simulink model "log_map_sl"  (Simulink 7.5)
settings: Solver=FixedStepDiscrete  StartTime=0.0  StopTime=50.0  FixedStep=0.1  RelTol=1e-3
values from neighbouring files (symbols this model uses):
  alpha = 0.2    [logmap_start.m]
  beta = 0.7    [logmap_start.m]
  lambda = 4.0    (= 4)    [logmap_start.m]
  y1_0 = 0.23421    [logmap_start.m]
  y2_0 = 0.86567    [logmap_start.m]
settings Model: OSC_ATGCV_WORKDIR=C:\test_ground\target_link_stuff\sixth\new_profile  Creator=alex  LastModifiedBy=alex
settings DataIOCC: LimitDataPoints=off  SaveOutput=off  SaveTime=off
settings OptimizationCC: BooleanDataType=off  InitFltsAndDblsToZero=on
settings DebuggingCC: SaveWithParameterizedLinksMsg=none  SignalResolutionControl=TryResolveAllWithWarning  SolverPrmCheckMsg=none  MultiTaskDSMMsg=warning  MultiTaskCondExecSysMsg=none  StrictBusMsg=None
settings HardwareCC: TargetUnknown=on
settings RTWCC: IncludeERTFirstTime=on
settings GRTTargetCC: TargetFcnLib=ansi_tfl_tmw.mat

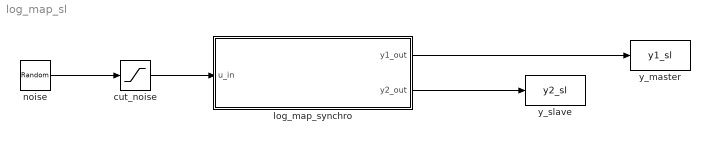
== system log_map_sl ==
  cut_noise : Saturate  UpperLimit=1  LowerLimit=0
  log_map_synchro : Subsystem
  noise : RandomNumber  Mean=0.5  SampleTime=0
  y_master : ToWorkspace  VariableName=y1_sl  SampleTime=-1  SaveFormat=Array
  y_slave : ToWorkspace  VariableName=y2_sl  SampleTime=-1  SaveFormat=Array
  wires:
  noise/1 -> cut_noise/1
  log_map_synchro/1(y1_out) -> y_master/1
  cut_noise/1 -> log_map_synchro/1(u_in)
  log_map_synchro/2(y2_out) -> y_slave/1

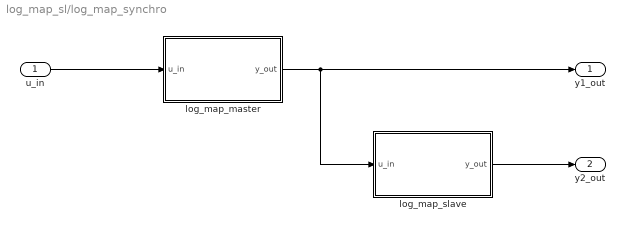
== system log_map_sl/log_map_synchro ==
  u_in : Inport  OutDataType=sfix(16)  OutScaling=2^0
  log_map_master : Subsystem
  log_map_slave : Subsystem
  y1_out : Outport  OutDataType=sfix(16)  OutScaling=2^0
  y2_out : Outport  Port=2  OutDataType=sfix(16)  OutScaling=2^0
  wires:
  u_in/1 -> log_map_master/1(u_in)
  log_map_master/1(y_out) -> y1_out/1, log_map_slave/1(u_in)
  log_map_slave/1(y_out) -> y2_out/1

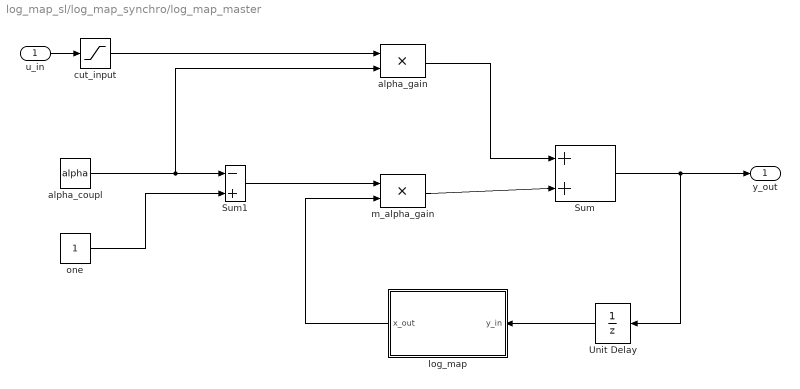
== system log_map_sl/log_map_synchro/log_map_master ==
  u_in : Inport  OutDataType=sfix(16)  OutScaling=2^0
  Sum : Sum  Inputs=+|+  OutDataType=sfix(16)  OutScaling=2^0  SaturateOnIntegerOverflow=on  InputSameDT=on  OutDataTypeStr=Inherit: Same as first input
  Sum1 : Sum  Inputs=-|+  OutDataType=sfix(16)  OutScaling=2^0  SaturateOnIntegerOverflow=on  InputSameDT=on  OutDataTypeStr=Inherit: Same as first input
  Unit Delay : UnitDelay  X0=y1_0  SampleTime=-1
  alpha_coupl : Constant  Value=alpha  OutDataType=sfix(16)  OutScaling=2^0
  alpha_gain : Product  OutDataType=sfix(16)  OutScaling=2^0  SaturateOnIntegerOverflow=on  RndMeth=Zero  InputSameDT=on  OutDataTypeStr=Inherit: Same as first input
  cut_input : Saturate  UpperLimit=1  LowerLimit=0
  log_map : Subsystem
  m_alpha_gain : Product  OutDataType=sfix(16)  OutScaling=2^0  SaturateOnIntegerOverflow=on  RndMeth=Zero  InputSameDT=on  OutDataTypeStr=Inherit: Same as first input
  one : Constant  OutDataType=sfix(16)  OutScaling=2^0
  y_out : Outport  OutDataType=sfix(16)  OutScaling=2^0
  wires:
  alpha_gain/1 -> Sum/1
  log_map/1(x_out) -> m_alpha_gain/2
  Sum/1 -> Unit Delay/1, y_out/1
  u_in/1 -> cut_input/1
  cut_input/1 -> alpha_gain/1
  Unit Delay/1 -> log_map/1(y_in)
  m_alpha_gain/1 -> Sum/2
  one/1 -> Sum1/2
  alpha_coupl/1 -> Sum1/1, alpha_gain/2
  Sum1/1 -> m_alpha_gain/1

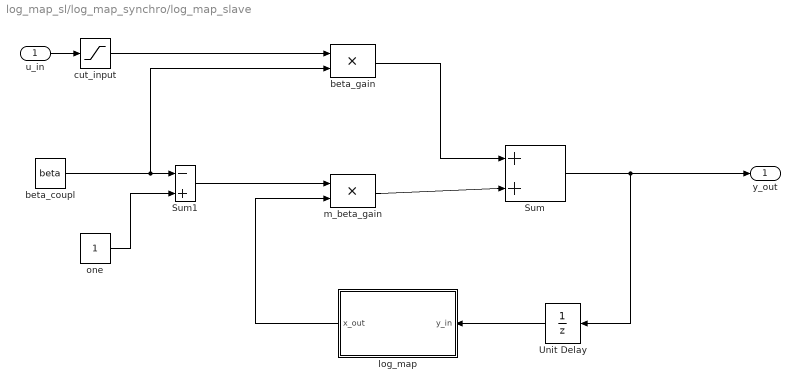
== system log_map_sl/log_map_synchro/log_map_slave ==
  u_in : Inport  OutDataType=sfix(16)  OutScaling=2^0
  Sum : Sum  Inputs=+|+  OutDataType=sfix(16)  OutScaling=2^0  SaturateOnIntegerOverflow=on  InputSameDT=on  OutDataTypeStr=Inherit: Same as first input
  Sum1 : Sum  Inputs=-|+  OutDataType=sfix(16)  OutScaling=2^0  SaturateOnIntegerOverflow=on  InputSameDT=on  OutDataTypeStr=Inherit: Same as first input
  Unit Delay : UnitDelay  X0=y2_0  SampleTime=-1
  beta_coupl : Constant  Value=beta  OutDataType=sfix(16)  OutScaling=2^0
  beta_gain : Product  OutDataType=sfix(16)  OutScaling=2^0  SaturateOnIntegerOverflow=on  RndMeth=Zero  InputSameDT=on  OutDataTypeStr=Inherit: Same as first input
  cut_input : Saturate  UpperLimit=1  LowerLimit=0
  log_map : Subsystem
  m_beta_gain : Product  OutDataType=sfix(16)  OutScaling=2^0  SaturateOnIntegerOverflow=on  RndMeth=Zero  InputSameDT=on  OutDataTypeStr=Inherit: Same as first input
  one : Constant  OutDataType=sfix(16)  OutScaling=2^0
  y_out : Outport  OutDataType=sfix(16)  OutScaling=2^0
  wires:
  m_beta_gain/1 -> Sum/2
  Unit Delay/1 -> log_map/1(y_in)
  cut_input/1 -> beta_gain/1
  u_in/1 -> cut_input/1
  Sum/1 -> y_out/1, Unit Delay/1
  log_map/1(x_out) -> m_beta_gain/2
  beta_gain/1 -> Sum/1
  Sum1/1 -> m_beta_gain/1
  beta_coupl/1 -> Sum1/1, beta_gain/2
  one/1 -> Sum1/2

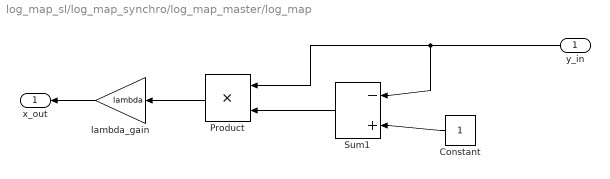
== system log_map_sl/log_map_synchro/log_map_master/log_map ==
  y_in : Inport  OutDataType=sfix(16)  OutScaling=2^0
  Constant : Constant  OutDataType=sfix(16)  OutScaling=2^0
  Product : Product  OutDataType=sfix(16)  OutScaling=2^0  SaturateOnIntegerOverflow=on  RndMeth=Zero  InputSameDT=on  OutDataTypeStr=Inherit: Same as first input
  Sum1 : Sum  Inputs=-|+  OutDataType=sfix(16)  OutScaling=2^0  SaturateOnIntegerOverflow=on  InputSameDT=on  OutDataTypeStr=Inherit: Same as first input
  lambda_gain : Gain  Gain=lambda  ParameterDataType=sfix(16)  ParameterScaling=2^0  OutDataType=sfix(16)  OutScaling=2^0  SaturateOnIntegerOverflow=on  OutDataTypeStr=Inherit: Same as input  ParamDataTypeStr=Inherit: Same as input
  x_out : Outport  OutDataType=sfix(16)  OutScaling=2^0
  wires:
  Constant/1 -> Sum1/2
  Sum1/1 -> Product/2
  y_in/1 -> Product/1, Sum1/1
  Product/1 -> lambda_gain/1
  lambda_gain/1 -> x_out/1

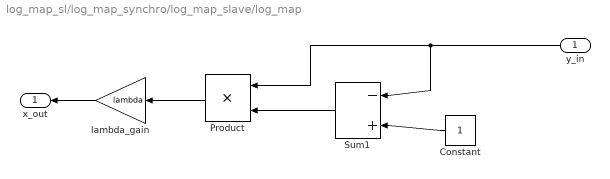
== system log_map_sl/log_map_synchro/log_map_slave/log_map ==
  y_in : Inport  OutDataType=sfix(16)  OutScaling=2^0
  Constant : Constant  OutDataType=sfix(16)  OutScaling=2^0
  Product : Product  OutDataType=sfix(16)  OutScaling=2^0  SaturateOnIntegerOverflow=on  RndMeth=Zero  InputSameDT=on  OutDataTypeStr=Inherit: Same as first input
  Sum1 : Sum  Inputs=-|+  OutDataType=sfix(16)  OutScaling=2^0  SaturateOnIntegerOverflow=on  InputSameDT=on  OutDataTypeStr=Inherit: Same as first input
  lambda_gain : Gain  Gain=lambda  ParameterDataType=sfix(16)  ParameterScaling=2^0  OutDataType=sfix(16)  OutScaling=2^0  SaturateOnIntegerOverflow=on  OutDataTypeStr=Inherit: Same as input  ParamDataTypeStr=Inherit: Same as input
  x_out : Outport  OutDataType=sfix(16)  OutScaling=2^0
  wires:
  lambda_gain/1 -> x_out/1
  Product/1 -> lambda_gain/1
  y_in/1 -> Sum1/1, Product/1
  Sum1/1 -> Product/2
  Constant/1 -> Sum1/2
